simulink model "ME598_R3_FinalProject_StateFlow"  (R2021b)
settings: Solver=ode23t  StartTime=0.0  StopTime=inf  RelTol=1e-3
InitFcn:
  | RPInit
model workspace (MAT data in the model file):
  mapForSim : object (value not decoded)
  occGrid : robotics.BinaryOccupancyGrid (value not decoded)
undefined symbols (not defined in the file): X, Y, Z
libraries: sm_lib x25, nesl_utility x11, RP_Simulator_Components x7, ME598_ProjectLibrary x3, RoboticsPlayground x2, Contact_Forces_Lib x2
(part 2 of 2)

== stateflow chart ME598_R3_FinalProject_StateFlow/Chart ==
  state ColorDetection1 [group]
    state Blue
      during:
      desiredAngle = calculateSlope(xPose, yPose, -2, 0);
      [leftMotor, rightMotor] = moveRobot(desiredAngle,tPose);
    state Green
      during:
      desiredAngle = calculateSlope(xPose, yPose, 2, -2);
      [leftMotor, rightMotor] = moveRobot(desiredAngle,tPose);
    state Red
      during:
      desiredAngle = calculateSlope(xPose, yPose, 2, 2);
      [leftMotor, rightMotor] = moveRobot(desiredAngle,tPose);
  state St2
    entry:
    leftMotor = 0;
    rightMotor = 0;
    st = 2;
    during:
    leftMotor = -120;
    rightMotor = -120;
  state St0
    entry:
    st = 0;
    leftMotor = 120;
    rightMotor = 120;
    during:
    desiredAngle = calculateSlope(xPose,yPose,0,1.5);
    [leftMotor, rightMotor] = moveRobot(desiredAngle, tPose);
  state St1
    entry:
    leftMotor = 0;
    rightMotor = 0;
    st = 1;
  state ColorDetection2 [group]
    state Blue
      during:
      desiredAngle = calculateSlope(xPose, yPose, -2, 0);
      [leftMotor, rightMotor] = moveRobot(desiredAngle,tPose);
    state Green
      during:
      desiredAngle = calculateSlope(xPose, yPose, 2, -2);
      [leftMotor, rightMotor] = moveRobot(desiredAngle,tPose);
    state Red
      during:
      desiredAngle = calculateSlope(xPose, yPose, 2, 2);
      [leftMotor, rightMotor] = moveRobot(desiredAngle,tPose);
  state stop
    entry: Stop =1;
  state Home
    entry:
    leftMotor = 0;
    rightMotor = 0;
    st = 10;
  state St3
    entry:
    leftMotor = 0;
    rightMotor = 0;
    st = 3;
    during:
    desiredAngle = calculateSlope(xPose, yPose, 0, -1.5);
    [leftMotor, rightMotor] = moveRobot(desiredAngle,tPose);
  state St5
    entry:
    leftMotor = 0;
    rightMotor = 0;
    st = 5;
    during:
    leftMotor = -120;
    rightMotor = -120;
  state St4
    entry:
    leftMotor = 0;
    rightMotor = 0;
    st = 4;
  state St6
    during:
    desiredAngle = calculateSlope(xPose, yPose, 0, 0);
    [leftMotor, rightMotor] = moveRobot(desiredAngle,tPose);
  ColorDetection1.Blue -> St2 : [xPose < -1.7 && yPose > -0.3 && yPose < 0.3]
  St1 -> ColorDetection1.Blue [order 1] : [isnan(rDist) && isnan(gDist) && ~isnan(bDist)]
  (default) -> St0
  St0 -> St1 : [xPose < 0.1 && xPose > -0.1 && yPose > 1.4 && yPose < 1.6]
  St1 -> ColorDetection1.Green [order 2] : [isnan(rDist) && ~isnan(gDist) && isnan(bDist)]
  ColorDetection1.Green -> St2 : [xPose > 1.7 && yPose < -1.7]
  St1 -> ColorDetection1.Red [order 3] : [~isnan(rDist) && isnan(gDist) && isnan(bDist)]
  Home -> stop : [st == 10]
  ColorDetection1.Red -> St2 : [xPose > 1.7 && yPose > 1.7]
  St2 -> St3 : [bDist >= 0.5 || gDist >= 0.5 || rDist >= 0.5]
  ColorDetection2.Blue -> St5 : [xPose < -1.7 && yPose > -0.3 && yPose < 0.3]
  St4 -> ColorDetection2.Blue [order 1] : [isnan(rDist) && isnan(gDist) && ~isnan(bDist)]
  St6 -> Home : [xPose < 0.1 && xPose > -0.1 && yPose < 0.1 && yPose > -0.1]
  ColorDetection2.Green -> St5 : [xPose > 1.7 && yPose < -1.7]
  St3 -> St4 : [xPose < 0.1 && xPose > -0.1 && yPose < -1.4 && yPose > -1.6]
  St4 -> ColorDetection2.Green [order 2] : [isnan(rDist) && ~isnan(gDist) && isnan(bDist)]
  St5 -> St6 : [bDist >= 0.5 || gDist >= 0.5 || rDist >= 0.5]
  ColorDetection2.Red -> St5 : [xPose > 1.7 && yPose > 1.7]
  St4 -> ColorDetection2.Red [order 3] : [~isnan(rDist) && isnan(gDist) && isnan(bDist)]
  data: x function_input; y function_input; xt function_input; yt function_input; targetAngle function_output; targetAngle function_input; tangentPose function_input; leftM function_output; rightM function_output; leftM function_output; rightM function_output; leftM function_output; rightM function_output; leftMotor output; rightMotor output; st local; desiredAngle local; yPose input; xPose input; rDist input; gDist input; bDist input; tPose input; left input; front input; right input; Stop local; stop output boolean
  function targetAngle = calculateSlope(x, y, xt, yt):
    | function targetAngle = calculateSlope(x, y, xt, yt)
    |         targetAngle = atan2d(yt-y, xt-x);
    | end
  function [leftM, rightM] = moveRobot(targetAngle,tangentPose):
    | function [leftM, rightM] = moveRobot(targetAngle,tangentPose)
    |         diff = tangentPose - targetAngle;
    |         if diff > 180
    |             diff = diff - 360;
    |         elseif diff < -180
    |             diff = diff + 360;
    |         end
    |         if diff < -10
    |             [leftM, rightM] = turnLeft();
    |         elseif diff > 10
    |             [leftM, rightM] = turnRight();
    |         % Wall avoidance algorithm. No matter where, if the wall is detected to be
    |         % near, the specific robot action is triggered.
    |         elseif front < 0.3
    |             if isnan(left) && isnan(right)
    |                 leftM = -120;
    |                 rightM = -120;
    |             elseif isnan(left) && ~isnan(right)
    |                 [leftM, rightM] = turnLeft();
    |             elseif ~isnan(left) && isnan(right)
    |                 [leftM, rightM] = turnRight();
    |             else
    |                 leftM = 120;
    |                 rightM = 120;
    |             end
    |         elseif right < 0.3 && isnan(left)
    |             [leftM, rightM] = turnLeft();
    |         elseif left < 0.3 && isnan(right)
    |             [leftM, rightM] = turnRight();
    |         else
    |             leftM = 120;
    |             rightM = 120;
    |         end
    | end
  function [leftM, rightM] = turnRight:
    | function [leftM, rightM] = turnRight()
    |         leftM = 60;
    |         rightM = -60;
    |     end
  function [leftM, rightM] = turnLeft:
    |  function [leftM, rightM] = turnLeft()
    |         leftM = -60;
    |         rightM = 60;
    |     end

== matlab function ME598_R3_FinalProject_StateFlow/-180* : 180* ==
  data: deg input; deg output
function deg = degWrap(deg)

% % Convert radians to degrees
% deg = 180/pi * rad;


% Wrap degree value to the range -180* : +180*
for idx = 1:length(deg)
    while deg(idx) < -180
        deg(idx) = deg(idx)+360;
    end
    
    while deg(idx) > 180
        deg(idx) = deg(idx)-360;
    end
end

return
